simulink model "firMatchedFilter"  (R2023b)
settings: Solver=FixedStepDiscrete  StartTime=0.0  StopTime=3  RelTol=1e-3
undefined symbols (not defined in the file): fmWave
libraries: dsparch4 x1, dspsrcs4 x1
settings Model: Creator=krsh  LastModifiedBy=krsh
settings SolverCC: AlgebraicLoopSolver=TrustRegion  AutoInsertRateTranBlk=on
settings DataIOCC: LimitDataPoints=on  SaveOutput=off  SignalLogging=off  SaveTime=off
settings OptimizationCC: ReuseModelBlockBuffer=off  LifeSpan=inf  SimCompilerOptimization=on
settings DebuggingCC: AlgebraicLoopMsg=error  SingleTaskRateTransMsg=error  UnconnectedInputMsg=warning  UnconnectedOutputMsg=warning  UnconnectedLineMsg=warning  AllowSymbolicDim=off  SubsystemReferenceDiagnosticForUnitTest=warning  SFUnexpectedBacktrackingDiag=warning  SFNoUnconditionalDefaultTransitionDiag=warning  SFExecutionAtInitializationDiag=none  ArithmeticOperatorsInVariantConditions=warning
settings ModelReferenceCC: EnableRefExpFcnMdlSchedulingChecks=on
settings SFSimCC: SimUseLocalCustomCode=off  CustomCodeUndefinedFunction=UseInterfaceOnly
settings RTWCC: RTWUseLocalCustomCode=off
settings CodeAppCC: StateflowObjectComments=on
settings GRTTargetCC: TargetLangStandard=C89/C90 (ANSI)
settings ConfigComp: CovMetricSettings=dw  CovSaveCumulativeToWorkspaceVar=on  CovSaveSingleToWorkspaceVar=on  CovExternalEMLEnable=off  CovSFcnEnable=off

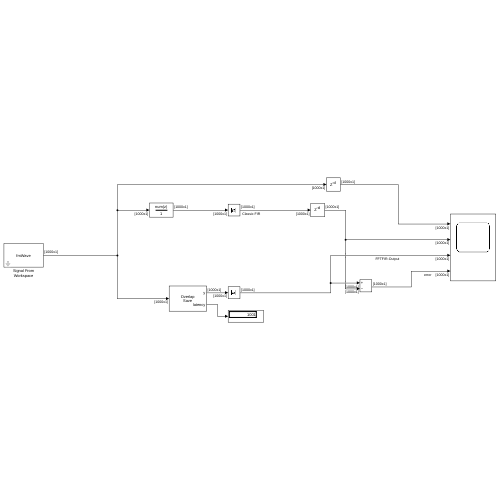
[thumbnail: Simulink's stored preview of the top-level diagram]
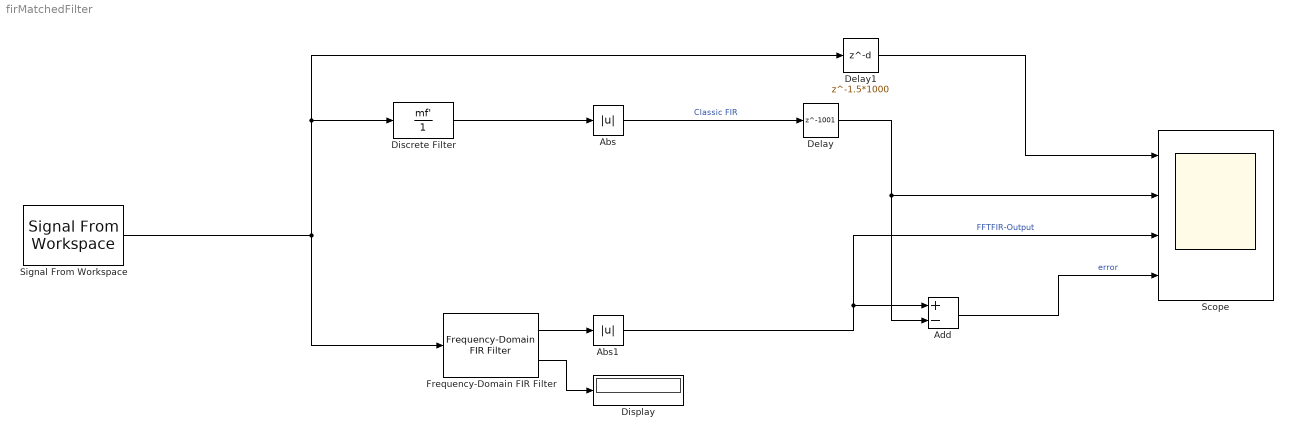
== system firMatchedFilter ==
  Abs : Abs  SaturateOnIntegerOverflow=off
  Abs1 : Abs  SaturateOnIntegerOverflow=off
  Add : Sum  Inputs=+-
  Delay : Delay  DelayLength=1001  InputProcessing=Columns as channels (frame based)
  Delay1 : Delay  DelayLength=1.5*1000  InputProcessing=Columns as channels (frame based)
  Discrete Filter : DiscreteFilter  Numerator=mf'  Denominator=1  InputProcessing=Columns as channels (frame based)
  Display : Display
  Frequency-Domain FIR Filter : dsparch4/Frequency-Domain FIR Filter  Method=Overlap-save  NumeratorDomain=Time  SpecifyNumeratorFromPort=off  SpecifyFrequencyResponseFromPort=off  FrequencyResponse=fft( fir1( 100, 0.3 ), 202 )  Numerator=mf'  PartitionForReducedLatency=off  NumeratorLength=101  InheritFFTLength=on  FFTLength=8192  PartitionLength=32  FilterIsReal=on  OutputFilterLatency=on  SimulateUsing=Code generation
  Scope : Scope  NumInputPorts=4
  Signal From Workspace : dspsrcs4/Signal From Workspace  X=fmWave  Ts=1/numel(fmWave)  nsamps=numel(fmWave)  OutputAfterFinalValue=Setting to zero  ignoreOrWarnInputAndFrameLengths=off  OutputFrames=off
  wires:
  Discrete Filter/1 -> Abs/1
  Abs/1 -> Delay/1  "Classic FIR"
  Frequency-Domain FIR Filter/1 -> Abs1/1
  Frequency-Domain FIR Filter/2 -> Display/1
  Abs1/1 -> Scope/3, Add/1  "FFTFIR-Output"
  Delay/1 -> Scope/2, Add/2
  Add/1 -> Scope/4  "error"
  Signal From Workspace/1 -> Delay1/1, Discrete Filter/1, Frequency-Domain FIR Filter/1
  Delay1/1 -> Scope/1
